simulink model "MLP_networks"  (Simulink 7.7)
settings: Solver=ode45  StartTime=0.0  StopTime=10.0  RelTol=1e-3
libraries: neural x1629
(part 37 of 39)

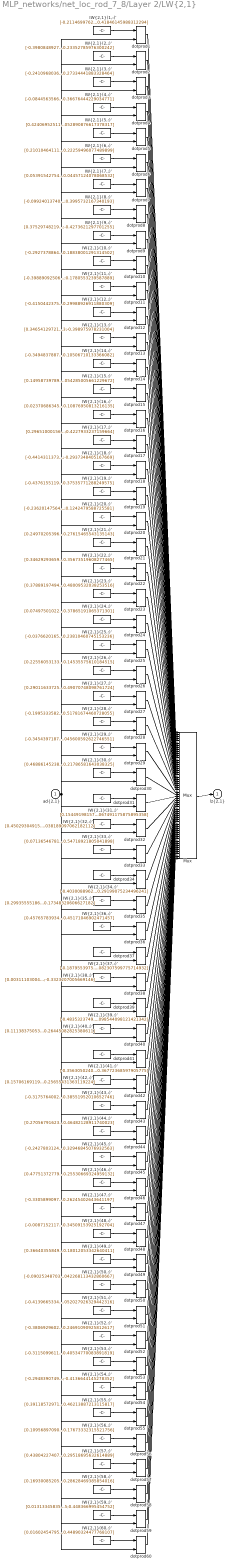
== system MLP_networks/net_loc_rod_7_8/Layer 2/LW{2,1} ==
  "ad{2,1}" : Inport  PortDimensions=30
      mask Display: e = 0.06;c1 = [120 230 180]/255;c2 = ([120 230 180]+0)/(256+128);c3 = ([120 230 180]+128)/(256+128);patch([0 1 1 0],[0 0 1 1],c1);patch([0 1 1 1-e 1-e 0+e],[0 0 1 1-e 0+e 0+e],c2);patch([0 0 1 1-e 0+e 0+e],[0 1 1 1-e 1-e 0+e],c3);plot([0 1 1 0 0],[0 0 1 1 0]);
  "IW{2,1}(1,:)'" : Constant  Value=[-0.21146997621039546;0.1787005268186822;-0.12752740467745058;0.016067071638450576;-0.12235408546227006;-0.17852808538274434;0.19905571302385183;-0.067136425730368585;-0.0067768321644114411;0.54870220483911258;-0.42020656081886343;-0.12598345099083619;-0.011990244863833863;0.6135444053346033;-0.4773668123338809;-0.193324856028015;0.10805389184329905;0.30099111362530301;-0.060658886408348836;-0.50358228920844961;0.1399816605193514;0.33527515805293134;-0.018501419259466748;-0.083532127652017438;-0.16727114040971849;-0.097846687438495311;0.67489377551507179;-0.15911273192774092;0.2018969122107295;0.41846145988312294]
      mask Display: e = 0.06;c1 = [120 150 230]/255;c2 = ([120 150 230]+0)/383;c3 = ([120 150 230]+128)/383;patch([0 1 1 0],[0 0 1 1],c1);patch([0 1 1 1-e 1-e 0+e],[0 0 1 1-e 0+e 0+e],c2);patch([0 0 1 1-e 0+e 0+e],[0 1 1 1-e 1-e 0+e],c3);plot([0 1 1 0 0],[0 0 1 1 0]);disp('weights');
  "IW{2,1}(10,:)'" : Constant  Value=[-0.29273788648906823;-0.037357828229991334;-0.22773890050256698;-0.30968530792614457;-0.49615165218394047;0.23606479405271147;0.40563509517156482;-0.29999824287545013;-0.17256378237103187;0.47126714664799529;0.44407619617747757;-0.10757485514139678;-0.17482857265268881;0.36671713821615326;-0.18080356771120096;0.065366586958579359;-0.14446083865181325;-0.17887743484563928;0.42734227596667446;0.28277330817400725;0.45515448634299227;0.071015480793099259;-0.28395197566194852;-0.1199493443662584;-0.40206922873751677;-0.48398371427401488;0.14944931358658167;0.11305211503756971;0.20456580456121731;0.18838001291314502]
      mask Display: e = 0.06;c1 = [120 150 230]/255;c2 = ([120 150 230]+0)/383;c3 = ([120 150 230]+128)/383;patch([0 1 1 0],[0 0 1 1],c1);patch([0 1 1 1-e 1-e 0+e],[0 0 1 1-e 0+e 0+e],c2);patch([0 0 1 1-e 0+e 0+e],[0 1 1 1-e 1-e 0+e],c3);plot([0 1 1 0 0],[0 0 1 1 0]);disp('weights');
  "IW{2,1}(11,:)'" : Constant  Value=[-0.39889092506138052;-0.4275835538017359;-0.32511150335896233;0.28892242676561714;0.45578651107884721;-0.18482022144359969;-0.22478669509114813;0.0049728433854331127;0.32363069467740652;0.27660248637856738;0.16076109133236791;-0.19624739030710531;0.29107209066212558;0.42889631806919265;-0.42019319304937902;0.12217366750246041;-0.20753927158064747;0.11793552922673974;-0.35871257984876376;-0.45565729203555694;-0.20211097382894469;0.13445461024557595;-0.45559456058637787;-0.2872597622686584;0.19453846433578159;0.14651978798851892;0.38826421370809849;-0.36396901889630989;0.126893114620279;0.1780553239587889]
      mask Display: e = 0.06;c1 = [120 150 230]/255;c2 = ([120 150 230]+0)/383;c3 = ([120 150 230]+128)/383;patch([0 1 1 0],[0 0 1 1],c1);patch([0 1 1 1-e 1-e 0+e],[0 0 1 1-e 0+e 0+e],c2);patch([0 0 1 1-e 0+e 0+e],[0 1 1 1-e 1-e 0+e],c3);plot([0 1 1 0 0],[0 0 1 1 0]);disp('weights');
  "IW{2,1}(12,:)'" : Constant  Value=[-0.41504423754284181;-0.10541864589245897;-0.26540642016952792;-0.45587397670798518;0.18174348321702438;-0.43639920630502216;0.17766944096707327;-0.070819957035922892;-0.0065499370473579037;-0.22376631232076638;0.22321247036835262;0.20806563057988148;0.34516832171771528;-0.39813588728048405;-0.023910453603159691;-0.376995339395851;0.50117640153788734;0.43143155357070445;-0.35559096132138468;-0.17720252487550822;0.36215683593358039;0.13278264773623732;-0.1679306990211975;-0.18550980248243978;0.25211556190080747;-0.081766191363968066;0.40832282582372692;0.29188924521375093;0.37245267681212951;0.29988926911880309]
      mask Display: e = 0.06;c1 = [120 150 230]/255;c2 = ([120 150 230]+0)/383;c3 = ([120 150 230]+128)/383;patch([0 1 1 0],[0 0 1 1],c1);patch([0 1 1 1-e 1-e 0+e],[0 0 1 1-e 0+e 0+e],c2);patch([0 0 1 1-e 0+e 0+e],[0 1 1 1-e 1-e 0+e],c3);plot([0 1 1 0 0],[0 0 1 1 0]);disp('weights');
  "IW{2,1}(13,:)'" : Constant  Value=[0.34654129721736626;0.058267335267196602;0.1313538573961211;0.32117851030304206;0.36847495399615338;-0.23014976872511941;0.050529159787372005;-0.41957233298420976;-0.50026376047860843;-0.21126161742055108;0.14440033170029823;0.39430411563634754;-0.29085490274842418;0.26110286689563839;0.25957262806243875;0.17722210166831831;-0.24353039310375968;0.29190478745005172;-0.11239084225195367;0.24214279601374994;0.49013648660364356;-0.3630262353329835;-0.25332860004283309;0.46643618745846277;-0.21049088759946574;0.2417603207200158;-0.086641971673878729;0.183659289252253;-0.26968673519371783;-0.398975978231004]
      mask Display: e = 0.06;c1 = [120 150 230]/255;c2 = ([120 150 230]+0)/383;c3 = ([120 150 230]+128)/383;patch([0 1 1 0],[0 0 1 1],c1);patch([0 1 1 1-e 1-e 0+e],[0 0 1 1-e 0+e 0+e],c2);patch([0 0 1 1-e 0+e 0+e],[0 1 1 1-e 1-e 0+e],c3);plot([0 1 1 0 0],[0 0 1 1 0]);disp('weights');
  "IW{2,1}(14,:)'" : Constant  Value=[-0.34948378874115515;-0.023285099402944136;-0.24155028029796627;-0.454197305691249;0.048690820381675722;-0.45668954148917057;-0.12386867710870801;0.31895266091835983;0.11654989402883481;-0.42928514627884645;0.35646698507237279;0.07392235321847955;-0.3544202289448779;-0.012334073195976843;-0.28129235836364991;-0.06313419786232756;0.51314505677168554;-0.17921688576145017;-0.46906937194239651;-0.38859415621423626;0.18638325501191114;0.4101400220760178;0.18648436250797576;0.15618621904718147;-0.24061558444086559;-0.59089612607543196;-0.086376071002519608;0.0071537225706980491;0.09694263837789667;0.10506710133366082]
      mask Display: e = 0.06;c1 = [120 150 230]/255;c2 = ([120 150 230]+0)/383;c3 = ([120 150 230]+128)/383;patch([0 1 1 0],[0 0 1 1],c1);patch([0 1 1 1-e 1-e 0+e],[0 0 1 1-e 0+e 0+e],c2);patch([0 0 1 1-e 0+e 0+e],[0 1 1 1-e 1-e 0+e],c3);plot([0 1 1 0 0],[0 0 1 1 0]);disp('weights');
  "IW{2,1}(15,:)'" : Constant  Value=[0.14958739789396006;-0.31622248358065086;0.44483975738123871;0.20581216107908121;0.058900059298798546;0.42472203063664044;0.37166274477279199;-0.1184907844980298;-0.051792612446473346;-0.39066281924433449;-0.43065735736006638;0.079180010700416956;0.099772926859170663;0.42027421305299018;-0.089487021769698583;-0.30661529746245508;-0.50027480396742263;-0.31162149611936302;-0.50403025978280724;0.414772031834998;0.41095291992449717;0.045553338512298806;0.1204591866567121;0.085487682293035286;0.087484996099007756;0.31535326519894413;0.27027444108721582;0.21696450715014592;0.27262312953604645;0.054285005661229672]
      mask Display: e = 0.06;c1 = [120 150 230]/255;c2 = ([120 150 230]+0)/383;c3 = ([120 150 230]+128)/383;patch([0 1 1 0],[0 0 1 1],c1);patch([0 1 1 1-e 1-e 0+e],[0 0 1 1-e 0+e 0+e],c2);patch([0 0 1 1-e 0+e 0+e],[0 1 1 1-e 1-e 0+e],c3);plot([0 1 1 0 0],[0 0 1 1 0]);disp('weights');
  "IW{2,1}(16,:)'" : Constant  Value=[0.023706863459614546;-0.081173148361446207;-0.50379262455104656;-0.077270292057569356;-0.46590027955644797;0.058990142536137539;0.32697862117578935;0.045460649668352365;-0.015377335766381249;0.40304473256424778;0.26045913009092447;0.23431451056562194;-0.40289434628235099;-0.26884057378781079;0.39012595962836205;-0.29533064252544122;-0.45481990030148284;-0.38757183019579888;-0.41397898555267076;0.20313722628997327;0.11263310335907406;0.012814103681988731;-0.26294490772119528;0.41438499706525977;0.11786525407351665;0.044017102963166278;0.013509758569270275;0.50229245674406764;0.44223057115010728;-0.10876950813216135]
      mask Display: e = 0.06;c1 = [120 150 230]/255;c2 = ([120 150 230]+0)/383;c3 = ([120 150 230]+128)/383;patch([0 1 1 0],[0 0 1 1],c1);patch([0 1 1 1-e 1-e 0+e],[0 0 1 1-e 0+e 0+e],c2);patch([0 0 1 1-e 0+e 0+e],[0 1 1 1-e 1-e 0+e],c3);plot([0 1 1 0 0],[0 0 1 1 0]);disp('weights');
  "IW{2,1}(17,:)'" : Constant  Value=[0.29651000156239232;0.0026098493922097447;-0.31953943439382587;0.34554121533590632;0.05540214075141308;0.37277415026173993;-0.48463650541833997;-0.25672931755785772;0.33052144400233996;0.1666639871413205;0.44775530632125926;0.35659233119910366;0.33407550787541501;-0.37966124343741503;0.23618498257497042;0.36986922205068196;-0.4219286014602705;0.054132804092709583;0.083858816482832929;-0.1731837624603603;0.057588761127868336;-0.16106115300339607;0.22592770573668322;0.13005759049709209;0.2898048870016911;-0.061150347510472866;0.17166922825824071;0.37126773464591079;0.43943168463761506;0.4227933237159664]
      mask Display: e = 0.06;c1 = [120 150 230]/255;c2 = ([120 150 230]+0)/383;c3 = ([120 150 230]+128)/383;patch([0 1 1 0],[0 0 1 1],c1);patch([0 1 1 1-e 1-e 0+e],[0 0 1 1-e 0+e 0+e],c2);patch([0 0 1 1-e 0+e 0+e],[0 1 1 1-e 1-e 0+e],c3);plot([0 1 1 0 0],[0 0 1 1 0]);disp('weights');
  "IW{2,1}(18,:)'" : Constant  Value=[-0.44143113730194228;0.17633715916815815;-0.37947672072661875;0.17238234258210028;0.46199742398370097;0.14227107755267548;-0.19319870014744228;-0.24715677063116889;-0.18227349664561876;0.30775389488483046;0.17020826092909741;0.21760471502795509;0.15522870117603071;0.2210633748262574;0.12410052758265187;0.31036194499484754;0.055824027131234827;0.44682738764117119;-0.026332294903917367;0.39764766556348113;0.30408777264186193;-0.40513414555727401;0.32453481356914388;0.17610087312841791;0.46487495034490439;-0.39806572759897774;-0.12453880132063784;-0.39285783194252838;0.21401787677834772;-0.2937348405167669]
      mask Display: e = 0.06;c1 = [120 150 230]/255;c2 = ([120 150 230]+0)/383;c3 = ([120 150 230]+128)/383;patch([0 1 1 0],[0 0 1 1],c1);patch([0 1 1 1-e 1-e 0+e],[0 0 1 1-e 0+e 0+e],c2);patch([0 0 1 1-e 0+e 0+e],[0 1 1 1-e 1-e 0+e],c3);plot([0 1 1 0 0],[0 0 1 1 0]);disp('weights');
  "IW{2,1}(19,:)'" : Constant  Value=[-0.43761551197607834;-0.38587229482789515;0.25308623894934063;-0.45503309969927086;-0.087023385864008262;-0.14290531807224027;0.0056304695619567094;-0.23592126459620547;-0.20166265784964943;0.47194329172266897;-0.20663531660181597;-0.27989136762347377;-0.078733274863598796;-0.3924182370338819;-0.19917857857779198;-0.089376444634931329;0.24387461702062602;0.37799652349479196;0.20422768593792315;-0.38809744765959464;0.33639882706800905;-0.26294526053579914;-0.27384288094928416;0.015235149817933615;-0.39716050055982155;-0.41500689935318691;0.24952595940176792;-0.071440152215982072;0.13154525989998689;0.37535771288249575]
      mask Display: e = 0.06;c1 = [120 150 230]/255;c2 = ([120 150 230]+0)/383;c3 = ([120 150 230]+128)/383;patch([0 1 1 0],[0 0 1 1],c1);patch([0 1 1 1-e 1-e 0+e],[0 0 1 1-e 0+e 0+e],c2);patch([0 0 1 1-e 0+e 0+e],[0 1 1 1-e 1-e 0+e],c3);plot([0 1 1 0 0],[0 0 1 1 0]);disp('weights');
  "IW{2,1}(2,:)'" : Constant  Value=[-0.3980848927449897;0.099767873376985713;0.055901671772898634;-0.18024564668432688;-0.38247266321365597;-0.18123431952774186;-0.066172527974077328;-0.2969408687944996;0.031568928497320591;0.080719321144406983;-0.42996544785748747;-0.1036629510086427;-0.40269917363255509;0.49699834900732426;-0.38722526252670075;-0.14583133531833165;0.32508107429993538;0.44787461284962349;-0.17531455739136875;0.36331316315674012;-0.10609522037081269;0.17702263708624641;-0.38673538446852879;-0.57788335383763423;-0.23571984709316041;0.18248327833894382;0.39885881271952595;0.063288733451592041;-0.012524785215832885;-0.23352785976300242]
      mask Display: e = 0.06;c1 = [120 150 230]/255;c2 = ([120 150 230]+0)/383;c3 = ([120 150 230]+128)/383;patch([0 1 1 0],[0 0 1 1],c1);patch([0 1 1 1-e 1-e 0+e],[0 0 1 1-e 0+e 0+e],c2);patch([0 0 1 1-e 0+e 0+e],[0 1 1 1-e 1-e 0+e],c3);plot([0 1 1 0 0],[0 0 1 1 0]);disp('weights');
  "IW{2,1}(20,:)'" : Constant  Value=[-0.23620147564937002;-0.47896139557275297;-0.34992652552263342;0.13845625998241173;-0.45402298719210155;-0.2396486568166207;0.41989404808606984;0.16334723517834743;-0.3177802426843796;-0.46979326795217097;0.38524572607480617;-0.069155346663146447;-0.30541592539321399;-0.47437998950672483;-0.35755383066865465;0.44491764240548493;-0.024597760319978051;0.48846134480745246;-0.18085549224212583;0.001992787326478852;0.12224998311299566;0.25410859306536876;0.088442779411769756;0.21625807065648439;0.2539480300281578;0.031984297498218496;0.055250884319854456;-0.029481525876926994;-0.27467430589790354;0.1242479588725581]
      mask Display: e = 0.06;c1 = [120 150 230]/255;c2 = ([120 150 230]+0)/383;c3 = ([120 150 230]+128)/383;patch([0 1 1 0],[0 0 1 1],c1);patch([0 1 1 1-e 1-e 0+e],[0 0 1 1-e 0+e 0+e],c2);patch([0 0 1 1-e 0+e 0+e],[0 1 1 1-e 1-e 0+e],c3);plot([0 1 1 0 0],[0 0 1 1 0]);disp('weights');
  "IW{2,1}(21,:)'" : Constant  Value=[0.24970205396266026;-0.30368452153875308;0.38960233122012744;0.39285232899465566;-0.31555962676973071;-0.41179211896315698;0.31532165051118149;0.26045694644665635;-0.35874053831330954;-0.248609902461498;0.38049425817967092;0.062756387848820705;0.24220950856737603;-0.0084194159354951947;-0.18038868926398749;-0.42792415841266668;0.43530201471787539;-0.030506943504887894;0.29383470722678451;0.18562016974043707;0.38056767871905789;0.22651091690967379;0.079323415444040646;-0.19821754349985082;0.1642595235926877;-0.028579143040850782;0.46443759219822744;-0.35319995118737973;0.35481360267634754;0.27615465543135143]
      mask Display: e = 0.06;c1 = [120 150 230]/255;c2 = ([120 150 230]+0)/383;c3 = ([120 150 230]+128)/383;patch([0 1 1 0],[0 0 1 1],c1);patch([0 1 1 1-e 1-e 0+e],[0 0 1 1-e 0+e 0+e],c2);patch([0 0 1 1-e 0+e 0+e],[0 1 1 1-e 1-e 0+e],c3);plot([0 1 1 0 0],[0 0 1 1 0]);disp('weights');
  "IW{2,1}(22,:)'" : Constant  Value=[0.34629293659256849;-0.34232392203635287;-0.39237341791955754;-0.47866264397780017;0.31102214686648072;0.085205427491816754;0.2272988845106941;-0.11865768458169609;0.01182977382122876;0.013024512480411737;-0.0043439585647598467;0.33094399048907852;-0.47012063031470169;-0.16031985020940576;-0.11538977776201249;0.18532309947608158;0.49701792644924286;0.10206413449444167;0.39857241678928734;-0.00054435816224695545;-0.31460234978150675;-0.3471735624267962;0.036943887440228203;0.076216590000834541;-0.12675005131727737;0.36900318284091932;0.32750947474346237;-0.45010485163695396;0.34015424692797258;0.35673519608277465]
      mask Display: e = 0.06;c1 = [120 150 230]/255;c2 = ([120 150 230]+0)/383;c3 = ([120 150 230]+128)/383;patch([0 1 1 0],[0 0 1 1],c1);patch([0 1 1 1-e 1-e 0+e],[0 0 1 1-e 0+e 0+e],c2);patch([0 0 1 1-e 0+e 0+e],[0 1 1 1-e 1-e 0+e],c3);plot([0 1 1 0 0],[0 0 1 1 0]);disp('weights');
  "IW{2,1}(23,:)'" : Constant  Value=[0.37889197494977922;0.46966046151556362;-0.058667266476898322;0.16867071573513395;-0.22247661854923267;-0.17575534222419759;0.0030651654324293414;0.40416026109470871;-0.17845055508212115;0.32153217832726022;-0.30200156621179236;-0.12860873292319935;-0.4772502125678435;-0.29147258144535554;-0.022980120945735087;-0.32154827138690989;-0.11816609082892754;-0.15910814564425224;0.025787575869094751;-0.38140341845561382;0.0056084789281396989;-0.25813567973061852;0.18332847675100045;-0.33499331661296217;-0.50220410171198193;-0.012841601619897476;-0.25877975814848692;0.34670138344482515;0.46323473383376385;0.48009532038253516]
      mask Display: e = 0.06;c1 = [120 150 230]/255;c2 = ([120 150 230]+0)/383;c3 = ([120 150 230]+128)/383;patch([0 1 1 0],[0 0 1 1],c1);patch([0 1 1 1-e 1-e 0+e],[0 0 1 1-e 0+e 0+e],c2);patch([0 0 1 1-e 0+e 0+e],[0 1 1 1-e 1-e 0+e],c3);plot([0 1 1 0 0],[0 0 1 1 0]);disp('weights');
  "IW{2,1}(24,:)'" : Constant  Value=[0.074975010226204938;-0.39560795465180898;-0.20016832609587551;0.029517363851006891;0.3882319885407795;-0.46162377855098002;-0.009094337137390723;-0.32288013520061459;-0.42043491047495002;-0.14388324273850953;0.3247253190110917;-0.43117257284360921;0.076592254477231766;0.21451395609055771;0.45407197922336817;-0.4735013615085622;-0.18161882995127179;0.26289697908279597;-0.38375772809776459;0.29199331972675124;0.30310102714024767;0.082971839586893512;0.11241473909256687;-0.093506693820450834;-0.20602873421321441;0.032509613790944768;0.18233951151772565;0.45609037806537084;0.24079301023929484;-0.37865191065371301]
      mask Display: e = 0.06;c1 = [120 150 230]/255;c2 = ([120 150 230]+0)/383;c3 = ([120 150 230]+128)/383;patch([0 1 1 0],[0 0 1 1],c1);patch([0 1 1 1-e 1-e 0+e],[0 0 1 1-e 0+e 0+e],c2);patch([0 0 1 1-e 0+e 0+e],[0 1 1 1-e 1-e 0+e],c3);plot([0 1 1 0 0],[0 0 1 1 0]);disp('weights');
  "IW{2,1}(25,:)'" : Constant  Value=[-0.037662016542426444;-0.35151344245318367;-0.1913758183606441;-0.3363771654809643;-0.31289048435707822;0.39346064692854854;-0.44629685540209563;0.051305724034052813;0.43075941194734624;-0.23981796082137449;-0.41816374692482805;0.2864305628583006;-0.26029853081317456;0.32170910971119954;-0.068258539521478229;0.099361550473145502;-0.29467220358681112;0.15751597104699339;0.3878390198216724;-0.16461461843008696;-0.38366616497494038;0.31193476506775053;0.47989412269386933;-0.45562466926037659;0.19708378460023931;-0.2970446978531846;0.13405844953042331;-0.1203899752078034;-0.022026506605086961;0.23810460745153236]
      mask Display: e = 0.06;c1 = [120 150 230]/255;c2 = ([120 150 230]+0)/383;c3 = ([120 150 230]+128)/383;patch([0 1 1 0],[0 0 1 1],c1);patch([0 1 1 1-e 1-e 0+e],[0 0 1 1-e 0+e 0+e],c2);patch([0 0 1 1-e 0+e 0+e],[0 1 1 1-e 1-e 0+e],c3);plot([0 1 1 0 0],[0 0 1 1 0]);disp('weights');
  "IW{2,1}(26,:)'" : Constant  Value=[0.22556053133794104;0.19878068824948267;-0.34435642162570818;0.14228013786976054;-0.1965267869481338;-0.545150861809231;0.1603163857033863;-0.37899032105463692;-0.12700165165527505;0.16372356897295565;-0.30987207481050993;0.15729553795603865;0.38155262481494728;-0.37950956520182205;-0.048847861874809793;-0.22513798673279042;-0.3872984081607565;0.24677125208404643;0.043727612517087504;0.054253048454819257;0.27746106883947674;0.060526773742849892;0.36432442393942194;0.29121129905918264;-0.4031788906670179;-0.48028066172554146;0.43868691910121921;-0.37220899392036438;-0.21782048237560606;0.14535575610184515]
      mask Display: e = 0.06;c1 = [120 150 230]/255;c2 = ([120 150 230]+0)/383;c3 = ([120 150 230]+128)/383;patch([0 1 1 0],[0 0 1 1],c1);patch([0 1 1 1-e 1-e 0+e],[0 0 1 1-e 0+e 0+e],c2);patch([0 0 1 1-e 0+e 0+e],[0 1 1 1-e 1-e 0+e],c3);plot([0 1 1 0 0],[0 0 1 1 0]);disp('weights');
  "IW{2,1}(27,:)'" : Constant  Value=[0.29011633725943087;0.3726387683248662;-0.45716179576096966;-0.27600463288060739;-0.17412213923411565;-0.27742772626975815;0.032725216793159886;0.28400389288287886;0.49168886461423555;-0.23104577525079187;0.41773720305610135;-0.0047213629109272561;0.47042378945695296;-0.15686079214693566;-0.0085423876417954382;0.43072872411871954;0.0047153130578263883;0.14562222436507721;0.12197855780342841;0.17517517809065392;-0.50849183443676216;0.1944614255514773;0.020399956783936905;-0.29078932122784085;-0.017599470433847752;-0.42480010799735735;0.2035574832654749;-0.068950168480692534;-0.31387861623877389;0.49070748098761724]
      mask Display: e = 0.06;c1 = [120 150 230]/255;c2 = ([120 150 230]+0)/383;c3 = ([120 150 230]+128)/383;patch([0 1 1 0],[0 0 1 1],c1);patch([0 1 1 1-e 1-e 0+e],[0 0 1 1-e 0+e 0+e],c2);patch([0 0 1 1-e 0+e 0+e],[0 1 1 1-e 1-e 0+e],c3);plot([0 1 1 0 0],[0 0 1 1 0]);disp('weights');
  "IW{2,1}(28,:)'" : Constant  Value=[-0.19953335828397756;0.1787340096775191;0.43535962465787664;-0.088748327120689155;0.18131651784988262;0.12683972101423385;0.2089418949989649;0.057451719740722849;-0.39498452225779856;-0.36985911925168063;-0.067234003913973522;-0.01361271317225117;0.43102062496152765;0.17228130578132919;-0.15941611711070178;-0.37896404594411848;-0.083475176706921075;0.13254501084806597;0.39222023890927887;-0.23758986991975978;-0.0018015657941055768;-0.46001049659044491;-0.25538243784813153;-0.56601809106139134;-0.43203662311795576;0.37641317747640296;-0.084784735356897151;-0.029009161020213666;0.38391304503138368;0.51781674460728055]
      mask Display: e = 0.06;c1 = [120 150 230]/255;c2 = ([120 150 230]+0)/383;c3 = ([120 150 230]+128)/383;patch([0 1 1 0],[0 0 1 1],c1);patch([0 1 1 1-e 1-e 0+e],[0 0 1 1-e 0+e 0+e],c2);patch([0 0 1 1-e 0+e 0+e],[0 1 1 1-e 1-e 0+e],c3);plot([0 1 1 0 0],[0 0 1 1 0]);disp('weights');
  "IW{2,1}(29,:)'" : Constant  Value=[-0.34543971879287205;-0.29489132074390234;-0.24696962803307826;0.49647510333907097;-0.40471964040815989;0.46437884000966578;-0.25277236125427549;0.30710242925501824;0.32059742932039131;-0.24667583704806467;0.45213739042058121;-0.27363708991078767;0.35960190599982161;0.18849551323594266;0.15639838442366785;0.35619265452036802;-0.26286605497825322;-0.41214854203658713;0.22154734887493349;-0.13138663205976536;-0.096047428252651293;0.27599393463425254;-0.080196998233805467;0.069400691344958576;0.11827441909794764;0.081778251520164047;0.47660542643447129;0.34208760101753183;-0.1119025785426609;0.045600592622746551]
      mask Display: e = 0.06;c1 = [120 150 230]/255;c2 = ([120 150 230]+0)/383;c3 = ([120 150 230]+128)/383;patch([0 1 1 0],[0 0 1 1],c1);patch([0 1 1 1-e 1-e 0+e],[0 0 1 1-e 0+e 0+e],c2);patch([0 0 1 1-e 0+e 0+e],[0 1 1 1-e 1-e 0+e],c3);plot([0 1 1 0 0],[0 0 1 1 0]);disp('weights');
  "IW{2,1}(3,:)'" : Constant  Value=[-0.24109680369356698;-0.12044948729027635;-0.3739822994948469;0.32637119658280994;0.5040702053153252;0.18462344409958908;-0.14778248932714283;0.26445054304919913;0.1961007232571387;0.03775375241135167;-0.50760161709712714;-0.28297499915067592;0.1395338155156052;-0.49642728934968355;0.47362181160356076;-0.30502701754001588;0.1843802482893924;0.40258489483549148;-0.3546959430913551;0.48470235853190186;0.18387960574992132;0.39629021339650494;0.16664759407004556;0.0059443414505693255;-0.076969682008419665;-0.1245541380212159;0.084890567373305789;0.13903255121441777;0.23744959974726421;-0.27334441883328464]
      mask Display: e = 0.06;c1 = [120 150 230]/255;c2 = ([120 150 230]+0)/383;c3 = ([120 150 230]+128)/383;patch([0 1 1 0],[0 0 1 1],c1);patch([0 1 1 1-e 1-e 0+e],[0 0 1 1-e 0+e 0+e],c2);patch([0 0 1 1-e 0+e 0+e],[0 1 1 1-e 1-e 0+e],c3);plot([0 1 1 0 0],[0 0 1 1 0]);disp('weights');
  "IW{2,1}(30,:)'" : Constant  Value=[0.46886145238061239;-0.46821195178826258;0.49757940597239614;-0.063678119441345549;0.20413044310338008;0.17361001813127278;-0.11631964214106998;-0.41734180788895564;0.059826488877993626;0.44434147143415886;-0.077295339659558371;0.28149373849567982;0.40915579802778351;-0.054934320707387158;0.41045065859799201;0.12223928574395884;0.15678496877759915;-0.18766420353004343;0.0061154992184617382;-0.09625036269833305;0.30951312134398334;0.48908454377933336;-0.23551386359797147;0.32352386328636551;-0.21464101574155647;0.41117005427710129;0.33207134015505146;-0.23649195581004753;-0.1099341556670177;-0.21786581643038325]
      mask Display: e = 0.06;c1 = [120 150 230]/255;c2 = ([120 150 230]+0)/383;c3 = ([120 150 230]+128)/383;patch([0 1 1 0],[0 0 1 1],c1);patch([0 1 1 1-e 1-e 0+e],[0 0 1 1-e 0+e 0+e],c2);patch([0 0 1 1-e 0+e 0+e],[0 1 1 1-e 1-e 0+e],c3);plot([0 1 1 0 0],[0 0 1 1 0]);disp('weights');
  "IW{2,1}(31,:)'" : Constant  Value=[0.15449198157872726;0.24586930824294537;-0.38800296230540471;0.40324649385257316;-0.3886816324683981;-0.36157325185069167;-0.37930109894984526;-0.3205378622766919;0.37995890996377663;-0.18607871614085089;0.24421054715412799;-0.29786996781175401;0.020560222499075687;0.4086200403736811;-0.1162903447661604;0.39077873841211419;-0.44440591003961621;0.33293875817486329;-0.27220772056374515;0.17790984114171568;0.29192235387250853;-0.14989635227563949;0.36457327132510492;0.24893664643231903;0.13146208001709514;-0.22884981331477094;0.37109227538268763;-0.40604667099263547;0.088513106567602723;0.0067491175875895358]
      mask Display: e = 0.06;c1 = [120 150 230]/255;c2 = ([120 150 230]+0)/383;c3 = ([120 150 230]+128)/383;patch([0 1 1 0],[0 0 1 1],c1);patch([0 1 1 1-e 1-e 0+e],[0 0 1 1-e 0+e 0+e],c2);patch([0 0 1 1-e 0+e 0+e],[0 1 1 1-e 1-e 0+e],c3);plot([0 1 1 0 0],[0 0 1 1 0]);disp('weights');
  "IW{2,1}(32,:)'" : Constant  Value=[0.45029304915694535;-0.51919504807781081;-0.39486383514527024;0.28794389007147753;-0.1773185276465486;-0.21254965834556955;-0.23180608538358763;-0.037246738524404591;-0.15648416300227402;0.14033531450354877;0.01993262937187493;0.44372072004745533;0.0032330387209468167;0.020135389201122934;0.18425608052372566;0.4978838725107908;0.11693169172204147;0.039229825820989522;0.4178439455765654;0.49472252892263913;-0.32480039178675518;0.20831734459238699;0.21787161857739443;-0.39854200725676692;-0.035942734169617553;0.48815469913645276;0.35789042401889526;0.34190100692954417;0.019073565245200125;0.038189097062182112]
      mask Display: e = 0.06;c1 = [120 150 230]/255;c2 = ([120 150 230]+0)/383;c3 = ([120 150 230]+128)/383;patch([0 1 1 0],[0 0 1 1],c1);patch([0 1 1 1-e 1-e 0+e],[0 0 1 1-e 0+e 0+e],c2);patch([0 0 1 1-e 0+e 0+e],[0 1 1 1-e 1-e 0+e],c3);plot([0 1 1 0 0],[0 0 1 1 0]);disp('weights');
  "IW{2,1}(33,:)'" : Constant  Value=[0.071365467818176473;0.33985114870666011;-0.30717118196814985;0.52419717135072608;0.15293515169914032;0.016211330291395175;0.25345111025069134;0.18795028788211271;0.41235231904195607;-0.18311317379285003;-0.45193333491083892;0.044943085669700567;0.20805154217645913;0.47061972979138028;-0.22980096377535286;0.08458310507934888;0.26853260968786558;-0.4397141683728002;0.037179617384346074;0.17754084013121657;0.1455434912226459;-0.35861560008750254;0.028207518541437517;0.36157036954018507;-0.063445329386757593;0.46860552411632744;0.11161922739802739;-0.24940697305740123;-0.15066912488949447;0.54718921805041898]
      mask Display: e = 0.06;c1 = [120 150 230]/255;c2 = ([120 150 230]+0)/383;c3 = ([120 150 230]+128)/383;patch([0 1 1 0],[0 0 1 1],c1);patch([0 1 1 1-e 1-e 0+e],[0 0 1 1-e 0+e 0+e],c2);patch([0 0 1 1-e 0+e 0+e],[0 1 1 1-e 1-e 0+e],c3);plot([0 1 1 0 0],[0 0 1 1 0]);disp('weights');
  "IW{2,1}(34,:)'" : Constant  Value=[-0.40300889622236463;0.29272058441593973;0.19581110140652544;-0.084766560557252624;0.46590590552974581;-0.33542127718590597;-0.17717978406555174;-0.29616833862899133;0.085593352405686607;0.30273649585132811;-0.29493974830012532;0.44257264518624007;0.23404878502144652;-0.070329754630065494;0.35480422830744751;-0.26553665522578213;0.052829357838023505;-0.14993548079997931;-0.31653499239892646;-0.25965754848776024;-0.21664232170386893;-0.004355836105473629;-0.40756962395525237;-0.25892110891927966;-0.054617321628751915;-0.3707564337806683;0.29957810503632987;0.49099044269358999;-0.41613978599325663;0.29199075234496241]
      mask Display: e = 0.06;c1 = [120 150 230]/255;c2 = ([120 150 230]+0)/383;c3 = ([120 150 230]+128)/383;patch([0 1 1 0],[0 0 1 1],c1);patch([0 1 1 1-e 1-e 0+e],[0 0 1 1-e 0+e 0+e],c2);patch([0 0 1 1-e 0+e 0+e],[0 1 1 1-e 1-e 0+e],c3);plot([0 1 1 0 0],[0 0 1 1 0]);disp('weights');
  "IW{2,1}(35,:)'" : Constant  Value=[0.29935555186089735;0.205482113194428;0.34252435432214323;0.24837060090996149;0.35368170277955685;-0.11238641520531181;0.0071817565571217499;0.36077721574436727;0.44858210308127849;-0.038219703007113123;-0.26227152906242723;0.43956460694593197;-0.09936670709139947;-0.11156899444224597;0.042643993988134156;-0.23028750688197525;0.40438940414544877;0.43083664674874406;0.27218208544591754;0.38454455668657123;0.31685591682136804;0.1672234980305691;0.11349246063697929;-0.49488780032403989;0.41075529341429995;0.27993988603064462;0.410676822270575;-0.020409616743587922;-0.23442054237324036;0.17348320606627182]
      mask Display: e = 0.06;c1 = [120 150 230]/255;c2 = ([120 150 230]+0)/383;c3 = ([120 150 230]+128)/383;patch([0 1 1 0],[0 0 1 1],c1);patch([0 1 1 1-e 1-e 0+e],[0 0 1 1-e 0+e 0+e],c2);patch([0 0 1 1-e 0+e 0+e],[0 1 1 1-e 1-e 0+e],c3);plot([0 1 1 0 0],[0 0 1 1 0]);disp('weights');
  "IW{2,1}(36,:)'" : Constant  Value=[0.45765783934650789;0.18891273220163241;0.068641574776556663;0.4135655856486305;-0.014618805821363316;-0.21420936293241227;-0.35706262805210071;0.20666133245794877;0.080518970346060301;-0.15844973988971314;0.38652329472732533;0.3660247219449676;-0.10983187195938007;0.028642894787803783;0.01350706399230551;0.38889182106538051;-0.022358446420009188;0.25215939268886595;-0.45831892498403842;-0.45753631861484756;0.39557741362981214;-0.29578158222602363;0.41110585208964007;0.0052195204793388092;-0.08111427886348474;-0.40290673639313862;0.26729706973803941;-0.35516932474995511;-0.43090520919794112;-0.45171046902471457]
      mask Display: e = 0.06;c1 = [120 150 230]/255;c2 = ([120 150 230]+0)/383;c3 = ([120 150 230]+128)/383;patch([0 1 1 0],[0 0 1 1],c1);patch([0 1 1 1-e 1-e 0+e],[0 0 1 1-e 0+e 0+e],c2);patch([0 0 1 1-e 0+e 0+e],[0 1 1 1-e 1-e 0+e],c3);plot([0 1 1 0 0],[0 0 1 1 0]);disp('weights');
  "IW{2,1}(37,:)'" : Constant  Value=[-0.18795539758381316;-0.33709817558575667;-0.10498168698472478;-0.33482484054882405;-0.4366930051593168;-0.27470556370003291;0.12481484009083957;-0.10788237006308318;-0.41657434180566411;-0.43355905446659176;-0.36209584465822914;0.3626134904425507;-0.034095997692807536;0.11315392452061304;0.35658927511848965;0.3346810927833298;0.0067726128351489022;-0.35060402338281876;-0.13343570061875407;0.41365753118713705;0.11021873120316128;-0.38360108679596716;0.31291520506926046;-0.34176202489483831;-0.3438230368627293;0.11022572460309817;-0.2342280557136599;-0.43829760529012368;-0.2335116857654142;-0.082307599775714932]
      mask Display: e = 0.06;c1 = [120 150 230]/255;c2 = ([120 150 230]+0)/383;c3 = ([120 150 230]+128)/383;patch([0 1 1 0],[0 0 1 1],c1);patch([0 1 1 1-e 1-e 0+e],[0 0 1 1-e 0+e 0+e],c2);patch([0 0 1 1-e 0+e 0+e],[0 1 1 1-e 1-e 0+e],c3);plot([0 1 1 0 0],[0 0 1 1 0]);disp('weights');
  "IW{2,1}(38,:)'" : Constant  Value=[0.0031110300449844336;0.1081444018278688;-0.42918127591925104;-0.01434167654595901;-0.43655714081879671;-0.39559809713947502;-0.091246781477109226;0.16690005273967223;-0.19002275965165558;-0.57036360723197921;0.23175032181094157;0.5824425209067281;0.43350113104492827;0.19041650178867772;0.41603160234274289;-0.21712278417308317;-0.5728708307955116;-0.015253874964726072;0.16659305773330715;-0.033248254645865498;0.024071091339402318;-0.41109408572933082;0.20994798982289897;-0.089636828876883248;0.026156740433248334;-0.23650691503810523;-0.046575420796282442;0.22150491152285176;-0.23979651649783915;-0.3323207005669146]
      mask Display: e = 0.06;c1 = [120 150 230]/255;c2 = ([120 150 230]+0)/383;c3 = ([120 150 230]+128)/383;patch([0 1 1 0],[0 0 1 1],c1);patch([0 1 1 1-e 1-e 0+e],[0 0 1 1-e 0+e 0+e],c2);patch([0 0 1 1-e 0+e 0+e],[0 1 1 1-e 1-e 0+e],c3);plot([0 1 1 0 0],[0 0 1 1 0]);disp('weights');
  "IW{2,1}(39,:)'" : Constant  Value=[-0.4835323749616523;0.31040278631905849;0.10047082836331186;-0.44502359853670193;0.39361966468221593;-0.34187227847267937;-0.18385257985250303;0.063961557191133347;-0.13311223909844291;-0.10037287921349862;-0.022734847026702414;0.32795556493781491;-0.20184661004759019;0.31043902538334567;0.48581448623302109;0.2923177940710513;-0.0082319895963805199;-0.23047279705256349;0.079154749884875836;-0.35425935283586912;-0.33585786795363404;0.55922628182483347;0.024927542637002982;-0.5369677098909581;-0.0095303478724389854;-0.21849709157034933;-0.21380711845089198;0.18488659257561837;0.37658112690975565;-0.098544098121421342]
      mask Display: e = 0.06;c1 = [120 150 230]/255;c2 = ([120 150 230]+0)/383;c3 = ([120 150 230]+128)/383;patch([0 1 1 0],[0 0 1 1],c1);patch([0 1 1 1-e 1-e 0+e],[0 0 1 1-e 0+e 0+e],c2);patch([0 0 1 1-e 0+e 0+e],[0 1 1 1-e 1-e 0+e],c3);plot([0 1 1 0 0],[0 0 1 1 0]);disp('weights');
  "IW{2,1}(4,:)'" : Constant  Value=[-0.084456356670670585;0.39332853492416614;-0.14093791023297814;-0.24699434973438217;0.037218999998135292;0.057290859811489341;-0.078827547784478064;0.49932008441699871;0.16387379971577443;-0.040748085545927626;-0.009324468468041516;-0.19160814023664818;-0.32053131109424393;-0.11908011228852317;-0.041753985083747211;0.26962081886530981;0.46929550230303646;-0.4728704361695264;0.068000938155538287;0.52995252288102757;-0.27876691608214754;0.34925409397203971;-0.023685241942146756;0.1027174484119477;-0.32882096042564896;0.5005590567264776;0.28540974607274233;-0.50723706812721148;0.21128315049192911;0.36676444229034771]
      mask Display: e = 0.06;c1 = [120 150 230]/255;c2 = ([120 150 230]+0)/383;c3 = ([120 150 230]+128)/383;patch([0 1 1 0],[0 0 1 1],c1);patch([0 1 1 1-e 1-e 0+e],[0 0 1 1-e 0+e 0+e],c2);patch([0 0 1 1-e 0+e 0+e],[0 1 1 1-e 1-e 0+e],c3);plot([0 1 1 0 0],[0 0 1 1 0]);disp('weights');
  "IW{2,1}(40,:)'" : Constant  Value=[0.11138375053922149;0.10725746152537521;-0.40441884661729288;-0.37853098423894987;-0.08157669713924344;-0.15157684402681071;0.028628353347344079;-0.43210093459350013;-0.44846964252056087;0.11118148102122939;0.1242481553642565;0.16879590214484513;0.41077554701764851;0.14755675464456003;0.21144023645213661;-0.20514570550553057;-0.44588331488494204;0.40541459720775785;-0.092804745325358151;-0.15342207436425032;0.097208902147965043;0.34979320899396732;0.33451829346632145;-0.16901843840161238;-0.39427988026929328;-0.36030296316647398;0.38700613792454092;-0.31771214900978895;-0.45420022589045494;-0.26445082825380611]
      mask Display: e = 0.06;c1 = [120 150 230]/255;c2 = ([120 150 230]+0)/383;c3 = ([120 150 230]+128)/383;patch([0 1 1 0],[0 0 1 1],c1);patch([0 1 1 1-e 1-e 0+e],[0 0 1 1-e 0+e 0+e],c2);patch([0 0 1 1-e 0+e 0+e],[0 1 1 1-e 1-e 0+e],c3);plot([0 1 1 0 0],[0 0 1 1 0]);disp('weights');
  "IW{2,1}(41,:)'" : Constant  Value=[-0.35630502406955966;-0.36974493824414606;0.15417390376028811;-0.38411362717766467;-0.35707706076629075;0.34165780337971213;0.14516683224012641;-0.21814421311647195;0.0032027169911279991;0.41624788464706797;-0.3397264421764124;-0.34898378374770811;-0.38215900969063754;-0.11404218518317454;-0.0050269406475612136;-0.098560432098857342;0.19486175046204038;0.32148116785508213;-0.38184911577693403;0.18293667936430713;-0.32949787704077893;0.35202275708123654;-0.36473945033324517;0.30077151631589694;0.2861707258441703;-0.080564081375307309;0.42006888197764058;0.11125025887557062;-0.24233566024583689;0.36772368597905775]
      mask Display: e = 0.06;c1 = [120 150 230]/255;c2 = ([120 150 230]+0)/383;c3 = ([120 150 230]+128)/383;patch([0 1 1 0],[0 0 1 1],c1);patch([0 1 1 1-e 1-e 0+e],[0 0 1 1-e 0+e 0+e],c2);patch([0 0 1 1-e 0+e 0+e],[0 1 1 1-e 1-e 0+e],c3);plot([0 1 1 0 0],[0 0 1 1 0]);disp('weights');
  "IW{2,1}(42,:)'" : Constant  Value=[0.15706169119829308;-0.34970464264246925;-0.091467553719374178;0.089096796137939638;0.37726052407804506;-0.45569306047604091;-0.40770262293161275;-0.23251625005436713;-0.25419916471996584;0.061556156981641227;0.38417584029606072;-0.20488679933615037;-0.11108397344155337;0.46208521453680423;-0.16681301652254793;0.009716834658453485;-0.31429738943502228;0.42058563389721992;0.39625395225088711;-0.32712238021736739;0.084481526805292709;-0.29846080219001225;0.07194158791340341;-0.47843218886833982;0.27604781968334097;0.087851162331685273;-0.42601946747014108;-0.17080271868571589;0.209081222714597;-0.25655431363119224]
      mask Display: e = 0.06;c1 = [120 150 230]/255;c2 = ([120 150 230]+0)/383;c3 = ([120 150 230]+128)/383;patch([0 1 1 0],[0 0 1 1],c1);patch([0 1 1 1-e 1-e 0+e],[0 0 1 1-e 0+e 0+e],c2);patch([0 0 1 1-e 0+e 0+e],[0 1 1 1-e 1-e 0+e],c3);plot([0 1 1 0 0],[0 0 1 1 0]);disp('weights');
  "IW{2,1}(43,:)'" : Constant  Value=[-0.31757640025894474;0.056653323308336612;-0.32544780806317231;0.3449113935863426;0.22500001165720365;0.066553259696957981;0.21248106162757274;0.096345459788785906;-0.34025605178291202;-0.44926824011835953;-0.33703884954801289;-0.39135850312812459;0.084811180139392969;0.29004102009119448;-0.066177614890907052;0.2824143243737593;-0.41299189747303039;0.23959623598881055;-0.36516527294692269;-0.029753147329238117;0.03851459755258807;-0.16463600865424638;0.2976532762799749;0.036542029343999097;0.44292641794603299;-0.31092484757236044;-0.14713729631980613;0.41061645318910794;-0.45692360248280139;0.38551952010652746]
      mask Display: e = 0.06;c1 = [120 150 230]/255;c2 = ([120 150 230]+0)/383;c3 = ([120 150 230]+128)/383;patch([0 1 1 0],[0 0 1 1],c1);patch([0 1 1 1-e 1-e 0+e],[0 0 1 1-e 0+e 0+e],c2);patch([0 0 1 1-e 0+e 0+e],[0 1 1 1-e 1-e 0+e],c3);plot([0 1 1 0 0],[0 0 1 1 0]);disp('weights');
  "IW{2,1}(44,:)'" : Constant  Value=[0.27056791623358634;0.08799096571828896;0.40404501597019188;0.22557856196010281;-0.24810705411037701;-0.46898974798625548;-0.48246857128286258;-0.018971563790798295;-0.14180175558241984;-0.11819502415132724;-0.26906558792700436;0.033084771748252563;0.49345840818175823;-0.38563447733884082;-0.24841433722989337;-0.20280384747095245;-0.35483187434085484;0.44982892766393817;0.14130516262448167;0.42433474138815308;-0.067420293627416056;-0.22114163016512606;-0.21059456031308763;-0.1947806306183705;0.082815646444673055;-0.25470852276293143;0.2875592759501811;0.39255425179318121;0.10175831647895807;-0.46482128911740023]
      mask Display: e = 0.06;c1 = [120 150 230]/255;c2 = ([120 150 230]+0)/383;c3 = ([120 150 230]+128)/383;patch([0 1 1 0],[0 0 1 1],c1);patch([0 1 1 1-e 1-e 0+e],[0 0 1 1-e 0+e 0+e],c2);patch([0 0 1 1-e 0+e 0+e],[0 1 1 1-e 1-e 0+e],c3);plot([0 1 1 0 0],[0 0 1 1 0]);disp('weights');
  "IW{2,1}(45,:)'" : Constant  Value=[-0.24278031243361256;0.16460435432975626;0.33695098142409952;-0.38763210309265494;0.11318182663408502;-0.24323292343715391;-0.35412139680927979;-0.48202397097123423;0.34298856029500091;0.45098885155589863;0.29640677932190812;0.12442504925656733;0.22785636922478969;-0.27471140977544156;-0.2568326759436787;-0.33040434674789931;0.40058542584282214;0.28838343142141509;-0.067936896110189549;-0.28159510671003796;0.078580146864540748;0.51250916638014188;0.32989365797735987;-0.26779269746604206;-0.255578957532062;-0.29727334764933683;0.13933585004022109;0.34436541155109002;-0.26846203565570803;-0.32946845076932563]
      mask Display: e = 0.06;c1 = [120 150 230]/255;c2 = ([120 150 230]+0)/383;c3 = ([120 150 230]+128)/383;patch([0 1 1 0],[0 0 1 1],c1);patch([0 1 1 1-e 1-e 0+e],[0 0 1 1-e 0+e 0+e],c2);patch([0 0 1 1-e 0+e 0+e],[0 1 1 1-e 1-e 0+e],c3);plot([0 1 1 0 0],[0 0 1 1 0]);disp('weights');
  "IW{2,1}(46,:)'" : Constant  Value=[0.47751372779563583;-0.004631941129258247;-0.26746797355239715;0.17883186503629808;-0.10548613834212665;0.13687902939422278;-0.40631954704837736;0.17093579645948126;0.095311678944684244;0.034110033251800002;0.3224740096213401;-0.15952180986137474;-0.31784651157245414;-0.45320379549388551;0.33045323818398969;0.22019799015671856;-0.35034858148840908;0.45625883071377721;-0.31719260036143726;-0.50139725511272237;0.1362457531355615;0.22618930416171001;-0.32470450433606052;-0.10633510402694961;-0.31408662865790887;-0.42624423653419202;0.15375441583054122;-0.12959182064022393;0.42217380252437764;-0.25530669324959132]
      mask Display: e = 0.06;c1 = [120 150 230]/255;c2 = ([120 150 230]+0)/383;c3 = ([120 150 230]+128)/383;patch([0 1 1 0],[0 0 1 1],c1);patch([0 1 1 1-e 1-e 0+e],[0 0 1 1-e 0+e 0+e],c2);patch([0 0 1 1-e 0+e 0+e],[0 1 1 1-e 1-e 0+e],c3);plot([0 1 1 0 0],[0 0 1 1 0]);disp('weights');
  "IW{2,1}(47,:)'" : Constant  Value=[-0.33058990973758129;-0.070122866651558854;-0.18964704315156067;0.15987361685157389;0.23026949273690664;0.44625637355610298;0.021772781753390227;-0.053731232580210356;0.08313635696579319;-0.35236494354447639;0.42953438289875867;0.075855817877353904;-0.39252730569594219;0.2648014400238784;0.33156686386675471;0.0039727953447689611;0.34232437544328292;0.42230368814878627;0.38625146824659068;0.37475339723843737;0.39234153591899412;-0.29576359594338791;0.044467362563895552;-0.18506463939778761;0.38881446230224065;-0.34300640961375639;0.31374053810287089;-0.40125736323329159;-0.07249681924861065;-0.26245402643641197]
      mask Display: e = 0.06;c1 = [120 150 230]/255;c2 = ([120 150 230]+0)/383;c3 = ([120 150 230]+128)/383;patch([0 1 1 0],[0 0 1 1],c1);patch([0 1 1 1-e 1-e 0+e],[0 0 1 1-e 0+e 0+e],c2);patch([0 0 1 1-e 0+e 0+e],[0 1 1 1-e 1-e 0+e],c3);plot([0 1 1 0 0],[0 0 1 1 0]);disp('weights');
  "IW{2,1}(48,:)'" : Constant  Value=[-0.0087152117694266774;-0.13863862046810108;0.43608461697351353;0.24508966048687675;-0.31744663574592236;0.037191100287168016;-0.0072845024835617401;0.14337407545120331;0.39230208708277053;-0.26769255922219354;-0.11432636796992721;-0.03563621621721013;-0.45920634652435793;-0.37383833599028848;-0.40166068602002503;-0.039420946924690912;0.47104501996266845;0.2893241869611558;-0.12079466381212473;-0.06437804183397336;-0.20116223091006691;0.19891379096875936;-0.31206785609352838;-0.43312577703778077;0.42758092973608697;-0.33646525622581219;-0.40853609113602746;-0.29060817876817463;-0.25084389770722287;0.34509153925192704]
      mask Display: e = 0.06;c1 = [120 150 230]/255;c2 = ([120 150 230]+0)/383;c3 = ([120 150 230]+128)/383;patch([0 1 1 0],[0 0 1 1],c1);patch([0 1 1 1-e 1-e 0+e],[0 0 1 1-e 0+e 0+e],c2);patch([0 0 1 1-e 0+e 0+e],[0 1 1 1-e 1-e 0+e],c3);plot([0 1 1 0 0],[0 0 1 1 0]);disp('weights');
  "IW{2,1}(49,:)'" : Constant  Value=[0.3664035584933632;0.067770670954671139;-0.50327300088757343;-0.34233762084274327;-0.35402379725705957;-0.19296107393069553;-0.1081773543595337;-0.16307479994707527;-0.4583418301479506;0.22467914290900112;-0.14833729870960458;-0.073885715771716473;-0.018165669962940525;-0.082222221434341144;0.060711633201345906;-0.066032059934777843;0.32062593551943042;-0.39250641268822206;-0.020872485141581968;0.4322512182315113;0.011773603078192489;0.49178856291556711;0.25916934822152971;0.37926759052257847;-0.0021654096910475704;0.15717470271648507;-0.20539255898025252;0.48579751391422438;0.53079080421219049;0.18012053342640411]
      mask Display: e = 0.06;c1 = [120 150 230]/255;c2 = ([120 150 230]+0)/383;c3 = ([120 150 230]+128)/383;patch([0 1 1 0],[0 0 1 1],c1);patch([0 1 1 1-e 1-e 0+e],[0 0 1 1-e 0+e 0+e],c2);patch([0 0 1 1-e 0+e 0+e],[0 1 1 1-e 1-e 0+e],c3);plot([0 1 1 0 0],[0 0 1 1 0]);disp('weights');
  "IW{2,1}(5,:)'" : Constant  Value=[0.42406952511844803;-0.44237375881799146;0.052029662046422891;-0.2036726275790991;-0.16138085114747366;-0.45866443703859072;0.42022368237748842;0.17880090432263859;0.21410679732378329;0.29083240625480378;-0.027317090467041123;0.16565705826923979;0.34867543373333398;0.36985335436086852;0.017207268552833648;0.16536654219096897;0.20655619520552929;0.26425984167836081;-0.22427098686588573;0.44797343941801077;-0.3670662051012662;-0.26225592994412833;0.10611024363293338;0.16269400333774611;0.38885702777445003;0.24951996685976113;-0.401400401142052;-0.34645210174152247;0.41358463544735835;0.0052890876617378317]
      mask Display: e = 0.06;c1 = [120 150 230]/255;c2 = ([120 150 230]+0)/383;c3 = ([120 150 230]+128)/383;patch([0 1 1 0],[0 0 1 1],c1);patch([0 1 1 1-e 1-e 0+e],[0 0 1 1-e 0+e 0+e],c2);patch([0 0 1 1-e 0+e 0+e],[0 1 1 1-e 1-e 0+e],c3);plot([0 1 1 0 0],[0 0 1 1 0]);disp('weights');
  "IW{2,1}(50,:)'" : Constant  Value=[-0.090253487030213214;0.081598635586078078;0.46147121846944167;-0.28886127677024581;0.33883489681456203;0.40165981324062394;-0.56466650847367117;0.40245104763383949;0.20615438894432719;-0.18197549865451798;0.016956460742601938;0.36270102368113011;-0.24568566434979652;0.36504064441923562;0.38856270937240456;-0.2600354429820021;0.14657922287302941;-0.041888408687903327;0.40638754651752573;-0.2321073116173509;-0.39567116183589202;0.33201864852183349;0.25861244614755802;-0.13658164572710443;-0.22688700876353052;0.36437012402211999;-0.36526649346534346;0.067317160225319389;-0.13567612251309988;-0.0042268113432860667]
      mask Display: e = 0.06;c1 = [120 150 230]/255;c2 = ([120 150 230]+0)/383;c3 = ([120 150 230]+128)/383;patch([0 1 1 0],[0 0 1 1],c1);patch([0 1 1 1-e 1-e 0+e],[0 0 1 1-e 0+e 0+e],c2);patch([0 0 1 1-e 0+e 0+e],[0 1 1 1-e 1-e 0+e],c3);plot([0 1 1 0 0],[0 0 1 1 0]);disp('weights');
  "IW{2,1}(51,:)'" : Constant  Value=[-0.41396653348116202;0.34481546560977799;-0.38370551468343417;-0.24768640312877804;-0.18676171803887764;0.084664044981117181;0.18188057084030662;-0.36349132386836369;0.33482426284392841;-0.27228810964946543;0.26642096315480446;-0.30463339503971015;0.43161924106555777;0.42743165422605561;-0.27882990713472916;0.21490073574264024;-0.4056956188624658;-0.32923050103717405;0.090698502245491544;-0.041262366321696824;0.41254424540788398;-0.30370897564739469;0.039541467367836106;0.17200596018618489;-0.26670037961120951;0.27133875503080035;-0.20835111014889679;-0.36281229977734114;-0.39168813383167578;0.052027926329442316]
      mask Display: e = 0.06;c1 = [120 150 230]/255;c2 = ([120 150 230]+0)/383;c3 = ([120 150 230]+128)/383;patch([0 1 1 0],[0 0 1 1],c1);patch([0 1 1 1-e 1-e 0+e],[0 0 1 1-e 0+e 0+e],c2);patch([0 0 1 1-e 0+e 0+e],[0 1 1 1-e 1-e 0+e],c3);plot([0 1 1 0 0],[0 0 1 1 0]);disp('weights');
  "IW{2,1}(52,:)'" : Constant  Value=[-0.38069296020580595;-0.37388677763221584;-0.43527438786809186;-0.10018933070750413;-0.4318270422538768;0.12392134299945326;0.37826031038383068;0.0091844734047052332;0.14314032290612055;-0.09244668315567818;-0.030740872675903589;0.41794729092759891;0.3527559533390181;-0.32905164889004118;-0.13743001235253696;0.3599498134481689;-0.46620731899696716;0.091515812358865661;0.01608888058031591;0.27662234577658446;0.32653038439819637;-0.20897341100774278;-0.3556822785121137;0.19019733497017738;0.18743268464084689;-0.42563891356459305;0.16643055557724315;0.15097951433225962;0.44754909421480576;0.24691090925812617]
      mask Display: e = 0.06;c1 = [120 150 230]/255;c2 = ([120 150 230]+0)/383;c3 = ([120 150 230]+128)/383;patch([0 1 1 0],[0 0 1 1],c1);patch([0 1 1 1-e 1-e 0+e],[0 0 1 1-e 0+e 0+e],c2);patch([0 0 1 1-e 0+e 0+e],[0 1 1 1-e 1-e 0+e],c3);plot([0 1 1 0 0],[0 0 1 1 0]);disp('weights');
  "IW{2,1}(53,:)'" : Constant  Value=[-0.31150996118461921;-0.27089022469089569;0.32394253167930198;-0.191332896808973;-0.047928062465361021;0.2168304813613636;0.41348417125848008;-0.26938956396830288;0.18050331556901592;-0.32919781355229311;0.11232928910461436;0.52365937693549347;0.42875880006211525;0.15022859047575604;0.3944117180161309;-0.41570133018361693;-0.16943344912310337;-0.20083450372814748;0.0097569727379068789;0.44711178267211388;0.14883499873980074;-0.25717842673559238;-0.4027557603667935;-0.50451607457401093;0.061209633399481662;-0.065048057934823808;0.29050523352105062;-0.13416195096729075;-0.058541334279196118;0.40534770083891819]
      mask Display: e = 0.06;c1 = [120 150 230]/255;c2 = ([120 150 230]+0)/383;c3 = ([120 150 230]+128)/383;patch([0 1 1 0],[0 0 1 1],c1);patch([0 1 1 1-e 1-e 0+e],[0 0 1 1-e 0+e 0+e],c2);patch([0 0 1 1-e 0+e 0+e],[0 1 1 1-e 1-e 0+e],c3);plot([0 1 1 0 0],[0 0 1 1 0]);disp('weights');
  "IW{2,1}(54,:)'" : Constant  Value=[-0.29483907497304479;0.2461652272708191;-0.3116494520304734;0.31512836122764426;0.31116596857941942;-0.34272257225836639;0.24982175491241396;-0.13851522175780689;0.4126703301849235;0.45388578747823;-0.19367576526746791;0.38149713324139073;-0.29411255446216084;-0.15238848125567891;-0.10514311756417806;0.38917047266746152;0.34756870536036333;-0.25814615700515281;0.18253749335206168;-0.15105768446019258;0.37290030345230779;-0.10436029482724127;0.088668445563039974;-0.35389946691784768;-0.072190366624104108;0.27381580640706399;0.32273906646128608;-0.11035444148249351;0.44508955593242322;-0.4136644145278352]
      mask Display: e = 0.06;c1 = [120 150 230]/255;c2 = ([120 150 230]+0)/383;c3 = ([120 150 230]+128)/383;patch([0 1 1 0],[0 0 1 1],c1);patch([0 1 1 1-e 1-e 0+e],[0 0 1 1-e 0+e 0+e],c2);patch([0 0 1 1-e 0+e 0+e],[0 1 1 1-e 1-e 0+e],c3);plot([0 1 1 0 0],[0 0 1 1 0]);disp('weights');
  "IW{2,1}(55,:)'" : Constant  Value=[0.39118572971401605;-0.2250950957472681;-0.20171941962608772;0.24447266606081422;0.42651138888792267;0.24439809411326288;-0.43758615906117754;0.037501986208607396;-0.15757758381644171;0.32632471546033442;0.067660957465974572;0.46099293780212147;0.46517367062536269;0.0041267922056686876;-0.49841771824710374;0.2969127225687424;-0.21344262901511921;0.30365400493615929;-0.11538990019070819;-0.092574669250930372;-0.093324047733008411;0.50712233899454184;-0.28998379619409087;0.2334155745609032;0.099475841957016961;0.055594834414815129;-0.0021604909246395665;0.25664450740436828;-0.29261847922183498;0.46213887213115817]
      mask Display: e = 0.06;c1 = [120 150 230]/255;c2 = ([120 150 230]+0)/383;c3 = ([120 150 230]+128)/383;patch([0 1 1 0],[0 0 1 1],c1);patch([0 1 1 1-e 1-e 0+e],[0 0 1 1-e 0+e 0+e],c2);patch([0 0 1 1-e 0+e 0+e],[0 1 1 1-e 1-e 0+e],c3);plot([0 1 1 0 0],[0 0 1 1 0]);disp('weights');
  "IW{2,1}(56,:)'" : Constant  Value=[0.10956897090519425;0.078067756651545819;-0.24671141335522642;-0.33721342820982447;-0.056033239765665509;0.41062236499752036;-0.39699099752884576;0.44969146015822581;0.44650051332625479;0.18436959306935513;0.19283016857168836;-0.28985513531977714;0.2116524262849116;0.10033481493051909;0.42138047710921517;-0.4703061900203232;0.14968360864179775;-0.11481193858597644;0.39424267411879671;0.34748191006008466;0.11095109673002851;-0.061238159900806902;0.40918527279530759;-0.22332485722843232;-0.01006708332520047;0.36222437450209882;0.46192024527265491;0.28260468344650974;0.18372450425154335;-0.17673332315521756]
      mask Display: e = 0.06;c1 = [120 150 230]/255;c2 = ([120 150 230]+0)/383;c3 = ([120 150 230]+128)/383;patch([0 1 1 0],[0 0 1 1],c1);patch([0 1 1 1-e 1-e 0+e],[0 0 1 1-e 0+e 0+e],c2);patch([0 0 1 1-e 0+e 0+e],[0 1 1 1-e 1-e 0+e],c3);plot([0 1 1 0 0],[0 0 1 1 0]);disp('weights');
  "IW{2,1}(57,:)'" : Constant  Value=[0.43804227407036861;-0.5159998225175878;-0.33701718762050747;-0.031017720500566372;-0.14871777161242183;0.10032211889922149;0.29063944480047055;0.25351143938520004;-0.035133259507619766;-0.056715336310332667;-0.40377197613044447;-0.14352543954831098;-0.35572455490944327;-0.44152754392004306;-0.31297546582117852;-0.50986311720027155;-0.24682890604361885;-0.43510966827534103;0.12548325502278765;-0.48710194909433746;-0.036590421752356751;-0.34184634242346773;-0.24358205861594248;-0.30545502383897483;-0.036095338360427061;0.26184896725401141;0.02401899745670423;-0.077217098911994936;0.025681641767577496;0.29518695632614889]
      mask Display: e = 0.06;c1 = [120 150 230]/255;c2 = ([120 150 230]+0)/383;c3 = ([120 150 230]+128)/383;patch([0 1 1 0],[0 0 1 1],c1);patch([0 1 1 1-e 1-e 0+e],[0 0 1 1-e 0+e 0+e],c2);patch([0 0 1 1-e 0+e 0+e],[0 1 1 1-e 1-e 0+e],c3);plot([0 1 1 0 0],[0 0 1 1 0]);disp('weights');
  "IW{2,1}(58,:)'" : Constant  Value=[0.16930085205123677;0.28371315035164307;-0.2470144855589633;0.21249229155357136;-0.0603844950946507;-0.39659481613133929;0.41014133912742501;-0.26557523198499799;-0.43504975054060191;0.39207545976322306;0.24260602150375118;0.42847675400455915;-0.095330919886004395;0.28464677983739034;0.1106155084756012;-0.46936152950406546;-0.28077973095678566;-0.3859824143681162;0.11270371019855152;0.06234339733511287;-0.078391991163682423;0.34866507362632232;0.050136422559474397;0.14960524205469086;0.3595381792035155;-0.44351990189113993;0.15651072103802235;0.22361535349654169;-0.42860118426337152;0.28628469385854016]
      mask Display: e = 0.06;c1 = [120 150 230]/255;c2 = ([120 150 230]+0)/383;c3 = ([120 150 230]+128)/383;patch([0 1 1 0],[0 0 1 1],c1);patch([0 1 1 1-e 1-e 0+e],[0 0 1 1-e 0+e 0+e],c2);patch([0 0 1 1-e 0+e 0+e],[0 1 1 1-e 1-e 0+e],c3);plot([0 1 1 0 0],[0 0 1 1 0]);disp('weights');
  "IW{2,1}(59,:)'" : Constant  Value=[0.013133458356596102;-0.16947000465113868;0.052525881261631262;-0.21148445095941876;-0.027816659817743623;-0.44765098287061333;0.27888652129112274;-0.19898294210082701;-0.44307614058338607;-0.47583075762891147;0.44927750716105758;0.38922229194838248;0.14808235883317414;-0.22702273786493946;0.1488214333108023;0.18174831869052846;0.11783905263004656;0.42033624531995128;-0.17774954126076445;-0.29596628040965173;0.43839517258557292;0.17122752653098278;-0.3024981661667504;0.12473123810865065;0.11513973250108625;-0.35313966621355009;-0.18685425840897918;0.1575305968009536;-0.49353159233018035;0.448366995454752]
      mask Display: e = 0.06;c1 = [120 150 230]/255;c2 = ([120 150 230]+0)/383;c3 = ([120 150 230]+128)/383;patch([0 1 1 0],[0 0 1 1],c1);patch([0 1 1 1-e 1-e 0+e],[0 0 1 1-e 0+e 0+e],c2);patch([0 0 1 1-e 0+e 0+e],[0 1 1 1-e 1-e 0+e],c3);plot([0 1 1 0 0],[0 0 1 1 0]);disp('weights');
  "IW{2,1}(6,:)'" : Constant  Value=[0.21010464111844185;0.12926919188583558;0.56291699377701754;0.14979898609763512;0.47705260514425762;0.20924330541288594;0.053979069364879659;-0.39148496782732456;0.18412309773327401;-0.052234674064068405;-0.077698218736815081;0.2576975729174994;0.079507111213841131;0.42250536873799344;0.28096110125392998;-0.25860390907989156;0.55715333238506881;0.061962856670715619;-0.2088604605645204;-0.32737400587205534;0.11548937129657158;0.28697672119984197;0.61540791806351858;-0.039176868476378648;0.011308823300464415;0.13052017253868084;0.40800611668465114;0.16259908279939292;0.052874027792722086;-0.22259496077489899]
      mask Display: e = 0.06;c1 = [120 150 230]/255;c2 = ([120 150 230]+0)/383;c3 = ([120 150 230]+128)/383;patch([0 1 1 0],[0 0 1 1],c1);patch([0 1 1 1-e 1-e 0+e],[0 0 1 1-e 0+e 0+e],c2);patch([0 0 1 1-e 0+e 0+e],[0 1 1 1-e 1-e 0+e],c3);plot([0 1 1 0 0],[0 0 1 1 0]);disp('weights');
  "IW{2,1}(60,:)'" : Constant  Value=[0.016024547959520175;0.30054613225487642;0.46819975932922692;0.32477253301061015;-0.24984846510593647;0.46239527413244885;-0.28380837242764628;-0.37452279222937757;-0.20947516667758992;0.27883915226055395;-0.12783456571549379;-0.021517592223803561;0.15516629139629934;-0.4411275155019645;0.3672365837654325;0.065536208012601863;0.24329959653357672;-0.38298854091379697;-0.32984530686665808;-0.31336203717149685;-0.051183133090782727;-0.461082886031706;0.28902583018536354;-0.19702489885207919;0.26932184312724489;0.069521434531048878;0.3471931958844186;0.033652027939839457;0.085705869417049496;-0.44890324477768107]
      mask Display: e = 0.06;c1 = [120 150 230]/255;c2 = ([120 150 230]+0)/383;c3 = ([120 150 230]+128)/383;patch([0 1 1 0],[0 0 1 1],c1);patch([0 1 1 1-e 1-e 0+e],[0 0 1 1-e 0+e 0+e],c2);patch([0 0 1 1-e 0+e 0+e],[0 1 1 1-e 1-e 0+e],c3);plot([0 1 1 0 0],[0 0 1 1 0]);disp('weights');
  "IW{2,1}(7,:)'" : Constant  Value=[0.053915427549097193;0.1596965522637947;0.26902295696116257;-0.17339342021059881;0.2606685104231774;0.32570238395898321;-0.055088312681813426;-0.27046632662772219;0.079876293089924791;0.35017269435133452;0.16710614151138262;0.31579823759025782;-0.29834439136182284;-0.18070985569978343;-0.52417852959924827;0.37108115940345238;-0.12263158364146902;-0.4246471823712164;0.47828974260846047;0.39908745108476446;-0.24859678324356294;0.44318829308833074;-0.27387169902745978;-0.2924361399575709;-0.50930123252806347;-0.33273751949952968;-0.036054405229582365;0.12998846643905893;0.035545257274345654;-0.04457124078068532]
      mask Display: e = 0.06;c1 = [120 150 230]/255;c2 = ([120 150 230]+0)/383;c3 = ([120 150 230]+128)/383;patch([0 1 1 0],[0 0 1 1],c1);patch([0 1 1 1-e 1-e 0+e],[0 0 1 1-e 0+e 0+e],c2);patch([0 0 1 1-e 0+e 0+e],[0 1 1 1-e 1-e 0+e],c3);plot([0 1 1 0 0],[0 0 1 1 0]);disp('weights');
  "IW{2,1}(8,:)'" : Constant  Value=[-0.099240137402005629;0.25878094886348363;-0.091868801042810727;-0.30135095888125585;-0.50449824652454511;0.34612873951193368;-0.0010664265809426621;-0.26419275822169624;0.12681942323158812;0.25130761519094069;-0.10613119039260542;-0.1210145857899538;-0.36209531488213426;0.43495748661332079;0.061338249665184169;-0.029357247193802553;0.13779394784072649;0.48322613101242501;0.14386863507301942;-0.09032181714271284;0.49079393686610273;0.12863720993809061;0.34622802166332106;-0.42898847754904523;0.33628940920755962;0.39121943936370257;-0.36796951538815104;-0.038054087692762743;-0.32171101554945147;0.3995732167340193]
      mask Display: e = 0.06;c1 = [120 150 230]/255;c2 = ([120 150 230]+0)/383;c3 = ([120 150 230]+128)/383;patch([0 1 1 0],[0 0 1 1],c1);patch([0 1 1 1-e 1-e 0+e],[0 0 1 1-e 0+e 0+e],c2);patch([0 0 1 1-e 0+e 0+e],[0 1 1 1-e 1-e 0+e],c3);plot([0 1 1 0 0],[0 0 1 1 0]);disp('weights');
  "IW{2,1}(9,:)'" : Constant  Value=[0.37529748219440684;-0.44796060268507837;-0.22584954532295556;-0.095751251308671001;-0.024323043282603866;0.06810181955577202;0.17947727422871981;-0.21143015007561128;0.45550926819454834;0.20387852971357945;-0.40495725927644266;-0.10068818474277683;-0.38347441272242178;-0.33955823499032295;0.24926485440558724;-0.045890003772746574;0.44145216905237583;-0.29324294209613544;-0.021654101945216501;-0.057536183337915776;0.33993952165605285;0.36454274439443385;0.19683473800907428;0.08663986345766006;0.32986231072661071;0.41235912278303605;-0.28620839531444137;0.46658941618340732;-0.029510303842826997;-0.4273621297701255]
      mask Display: e = 0.06;c1 = [120 150 230]/255;c2 = ([120 150 230]+0)/383;c3 = ([120 150 230]+128)/383;patch([0 1 1 0],[0 0 1 1],c1);patch([0 1 1 1-e 1-e 0+e],[0 0 1 1-e 0+e 0+e],c2);patch([0 0 1 1-e 0+e 0+e],[0 1 1 1-e 1-e 0+e],c3);plot([0 1 1 0 0],[0 0 1 1 0]);disp('weights');
  Mux : Mux  Inputs=60
      mask Display: e = 0.06;c1 = [120 150 230]/255;c2 = ([120 150 230]+0)/383;c3 = ([120 150 230]+128)/383;patch([0 1 1 0],[0 0 1 1],c1);patch([0 1 1 1-e 1-e 0+e],[0 0 1 1-e 0+e 0+e],c2);patch([0 0 1 1-e 0+e 0+e],[0 1 1 1-e 1-e 0+e],c3);plot([0 1 1 0 0],[0 0 1 1 0]);disp('Mux');
  dotprod{1..60} (60 alike) : neural/Weight Functions/dotprod  SystemSampleTime=-1
  "lz{2,1}" : Outport
      mask Display: e = 0.06;c1 = [120 230 180]/255;c2 = ([120 230 180]+0)/(256+128);c3 = ([120 230 180]+128)/(256+128);patch([0 1 1 0],[0 0 1 1],c1);patch([0 1 1 1-e 1-e 0+e],[0 0 1 1-e 0+e 0+e],c2);patch([0 0 1 1-e 0+e 0+e],[0 1 1 1-e 1-e 0+e],c3);plot([0 1 1 0 0],[0 0 1 1 0]);
  wires:
  "IW{2,1}(1,:)'"/1 -> dotprod1/1
  "ad{2,1}"/1 -> dotprod1/2, dotprod2/2, dotprod3/2, dotprod4/2, dotprod5/2, dotprod6/2, dotprod7/2, dotprod8/2, dotprod9/2, dotprod10/2, dotprod11/2, dotprod12/2, dotprod13/2, dotprod14/2, dotprod15/2, dotprod16/2, dotprod17/2, dotprod18/2, dotprod19/2, dotprod20/2, dotprod21/2, dotprod22/2, dotprod23/2, dotprod24/2, dotprod25/2, dotprod26/2, dotprod27/2, dotprod28/2, dotprod29/2, dotprod30/2, dotprod31/2, dotprod32/2, dotprod33/2, dotprod34/2, dotprod35/2, dotprod36/2, dotprod37/2, dotprod38/2, dotprod39/2, dotprod40/2, dotprod41/2, dotprod42/2, dotprod43/2, dotprod44/2, dotprod45/2, dotprod46/2, dotprod47/2, dotprod48/2, dotprod49/2, dotprod50/2, dotprod51/2, dotprod52/2, dotprod53/2, dotprod54/2, dotprod55/2, dotprod56/2, dotprod57/2, dotprod58/2, dotprod59/2, dotprod60/2
  dotprod1/1 -> Mux/1
  "IW{2,1}(2,:)'"/1 -> dotprod2/1
  dotprod2/1 -> Mux/2
  "IW{2,1}(3,:)'"/1 -> dotprod3/1
  dotprod3/1 -> Mux/3
  "IW{2,1}(4,:)'"/1 -> dotprod4/1
  dotprod4/1 -> Mux/4
  "IW{2,1}(5,:)'"/1 -> dotprod5/1
  dotprod5/1 -> Mux/5
  "IW{2,1}(6,:)'"/1 -> dotprod6/1
  dotprod6/1 -> Mux/6
  "IW{2,1}(7,:)'"/1 -> dotprod7/1
  dotprod7/1 -> Mux/7
  "IW{2,1}(8,:)'"/1 -> dotprod8/1
  dotprod8/1 -> Mux/8
  "IW{2,1}(9,:)'"/1 -> dotprod9/1
  dotprod9/1 -> Mux/9
  "IW{2,1}(10,:)'"/1 -> dotprod10/1
  dotprod10/1 -> Mux/10
  "IW{2,1}(11,:)'"/1 -> dotprod11/1
  dotprod11/1 -> Mux/11
  "IW{2,1}(12,:)'"/1 -> dotprod12/1
  dotprod12/1 -> Mux/12
  "IW{2,1}(13,:)'"/1 -> dotprod13/1
  dotprod13/1 -> Mux/13
  "IW{2,1}(14,:)'"/1 -> dotprod14/1
  dotprod14/1 -> Mux/14
  "IW{2,1}(15,:)'"/1 -> dotprod15/1
  dotprod15/1 -> Mux/15
  "IW{2,1}(16,:)'"/1 -> dotprod16/1
  dotprod16/1 -> Mux/16
  "IW{2,1}(17,:)'"/1 -> dotprod17/1
  dotprod17/1 -> Mux/17
  "IW{2,1}(18,:)'"/1 -> dotprod18/1
  dotprod18/1 -> Mux/18
  "IW{2,1}(19,:)'"/1 -> dotprod19/1
  dotprod19/1 -> Mux/19
  "IW{2,1}(20,:)'"/1 -> dotprod20/1
  dotprod20/1 -> Mux/20
  "IW{2,1}(21,:)'"/1 -> dotprod21/1
  dotprod21/1 -> Mux/21
  "IW{2,1}(22,:)'"/1 -> dotprod22/1
  dotprod22/1 -> Mux/22
  "IW{2,1}(23,:)'"/1 -> dotprod23/1
  dotprod23/1 -> Mux/23
  "IW{2,1}(24,:)'"/1 -> dotprod24/1
  dotprod24/1 -> Mux/24
  "IW{2,1}(25,:)'"/1 -> dotprod25/1
  dotprod25/1 -> Mux/25
  "IW{2,1}(26,:)'"/1 -> dotprod26/1
  dotprod26/1 -> Mux/26
  "IW{2,1}(27,:)'"/1 -> dotprod27/1
  dotprod27/1 -> Mux/27
  "IW{2,1}(28,:)'"/1 -> dotprod28/1
  dotprod28/1 -> Mux/28
  "IW{2,1}(29,:)'"/1 -> dotprod29/1
  dotprod29/1 -> Mux/29
  "IW{2,1}(30,:)'"/1 -> dotprod30/1
  dotprod30/1 -> Mux/30
  "IW{2,1}(31,:)'"/1 -> dotprod31/1
  dotprod31/1 -> Mux/31
  "IW{2,1}(32,:)'"/1 -> dotprod32/1
  dotprod32/1 -> Mux/32
  "IW{2,1}(33,:)'"/1 -> dotprod33/1
  dotprod33/1 -> Mux/33
  "IW{2,1}(34,:)'"/1 -> dotprod34/1
  dotprod34/1 -> Mux/34
  "IW{2,1}(35,:)'"/1 -> dotprod35/1
  dotprod35/1 -> Mux/35
  "IW{2,1}(36,:)'"/1 -> dotprod36/1
  dotprod36/1 -> Mux/36
  "IW{2,1}(37,:)'"/1 -> dotprod37/1
  dotprod37/1 -> Mux/37
  "IW{2,1}(38,:)'"/1 -> dotprod38/1
  dotprod38/1 -> Mux/38
  "IW{2,1}(39,:)'"/1 -> dotprod39/1
  dotprod39/1 -> Mux/39
  "IW{2,1}(40,:)'"/1 -> dotprod40/1
  dotprod40/1 -> Mux/40
  "IW{2,1}(41,:)'"/1 -> dotprod41/1
  dotprod41/1 -> Mux/41
  "IW{2,1}(42,:)'"/1 -> dotprod42/1
  dotprod42/1 -> Mux/42
  "IW{2,1}(43,:)'"/1 -> dotprod43/1
  dotprod43/1 -> Mux/43
  "IW{2,1}(44,:)'"/1 -> dotprod44/1
  dotprod44/1 -> Mux/44
  "IW{2,1}(45,:)'"/1 -> dotprod45/1
  dotprod45/1 -> Mux/45
  "IW{2,1}(46,:)'"/1 -> dotprod46/1
  dotprod46/1 -> Mux/46
  "IW{2,1}(47,:)'"/1 -> dotprod47/1
  dotprod47/1 -> Mux/47
  "IW{2,1}(48,:)'"/1 -> dotprod48/1
  dotprod48/1 -> Mux/48
  "IW{2,1}(49,:)'"/1 -> dotprod49/1
  dotprod49/1 -> Mux/49
  "IW{2,1}(50,:)'"/1 -> dotprod50/1
  dotprod50/1 -> Mux/50
  "IW{2,1}(51,:)'"/1 -> dotprod51/1
  dotprod51/1 -> Mux/51
  "IW{2,1}(52,:)'"/1 -> dotprod52/1
  dotprod52/1 -> Mux/52
  "IW{2,1}(53,:)'"/1 -> dotprod53/1
  dotprod53/1 -> Mux/53
  "IW{2,1}(54,:)'"/1 -> dotprod54/1
  dotprod54/1 -> Mux/54
  "IW{2,1}(55,:)'"/1 -> dotprod55/1
  dotprod55/1 -> Mux/55
  "IW{2,1}(56,:)'"/1 -> dotprod56/1
  dotprod56/1 -> Mux/56
  "IW{2,1}(57,:)'"/1 -> dotprod57/1
  dotprod57/1 -> Mux/57
  "IW{2,1}(58,:)'"/1 -> dotprod58/1
  dotprod58/1 -> Mux/58
  "IW{2,1}(59,:)'"/1 -> dotprod59/1
  dotprod59/1 -> Mux/59
  "IW{2,1}(60,:)'"/1 -> dotprod60/1
  dotprod60/1 -> Mux/60
  Mux/1 -> "lz{2,1}"/1
